simulink model "day3_TuNT54"  (R2017b)
settings: Solver=FixedStepAuto  StartTime=0.0  StopTime=1  FixedStep=0.002  RelTol=1e-3
libraries: simulink x5
settings Model: Creator=Admin  LastModifiedBy=Admin

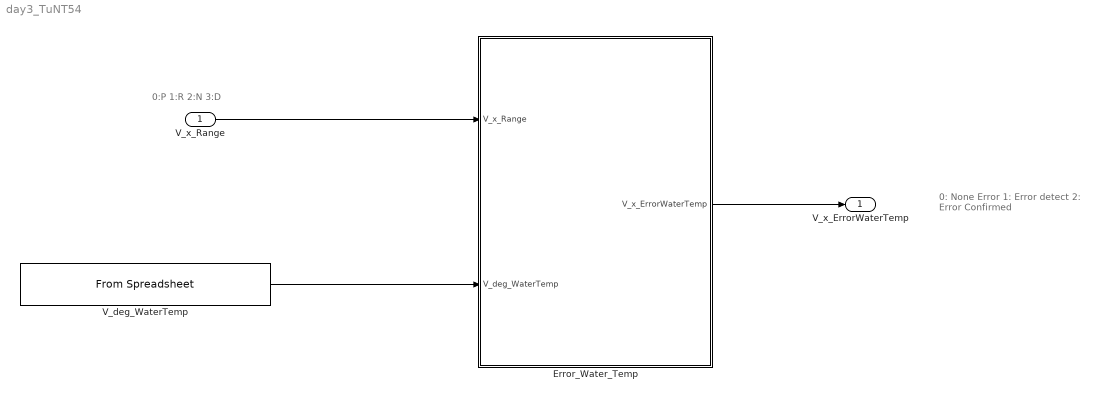
== system day3_TuNT54 ==
  note: 0: None Error
      | 1: Error detect
      | 2: Error Confirmed
  note: 0:P
      | 1:R
      | 2:N
      | 3:D
  V_x_Range : Inport
  Error_Water_Temp : Subsystem
  V_deg_WaterTemp : FromSpreadsheet  FileName=Data.xlsx
  V_x_ErrorWaterTemp : Outport
  wires:
  V_deg_WaterTemp/1 -> Error_Water_Temp/2(V_deg_WaterTemp)
  Error_Water_Temp/1(V_x_ErrorWaterTemp) -> V_x_ErrorWaterTemp/1
  V_x_Range/1 -> Error_Water_Temp/1(V_x_Range)

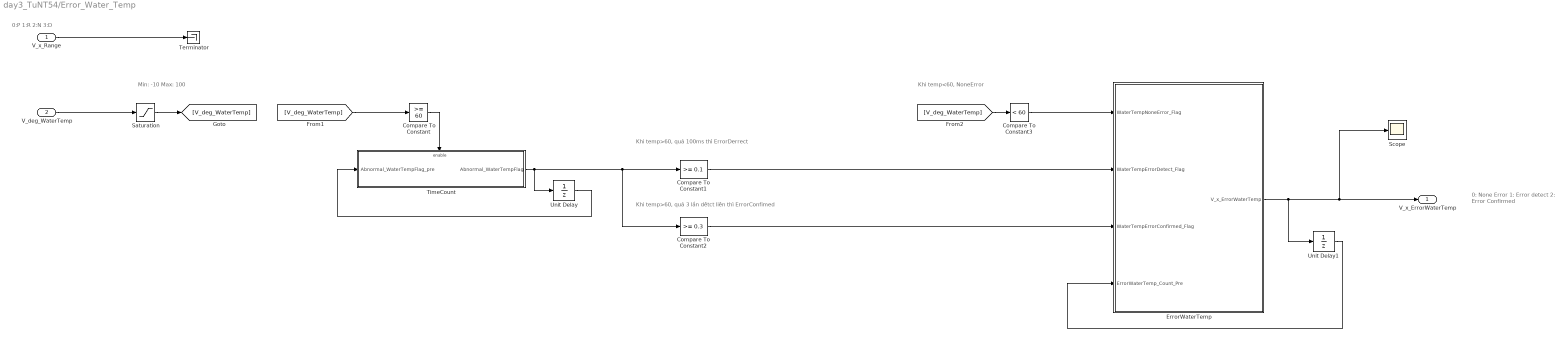
== system day3_TuNT54/Error_Water_Temp ==
  note: 0:P
      | 1:R
      | 2:N
      | 3:D
  note: 0: None Error
      | 1: Error detect
      | 2: Error Confirmed
  note: Min: -10
      | Max: 100
  note: Khi temp>60, quá 100ms thì ErrorDerrect
  note: Khi temp>60, quá 3 lần dêtct liên thì ErrorConfimed
  note: Khi temp<60, NoneError
  V_x_Range : Inport
  V_deg_WaterTemp : Inport  Port=2
  Compare To Constant : simulink/Logic and Bit Operations/Compare To Constant  relop=>=  const=60  OutDataTypeStr=boolean
  Compare To Constant1 : simulink/Logic and Bit Operations/Compare To Constant  relop=>=  const=0.1  OutDataTypeStr=boolean
  Compare To Constant2 : simulink/Logic and Bit Operations/Compare To Constant  relop=>=  const=0.3  OutDataTypeStr=boolean
  Compare To Constant3 : simulink/Logic and Bit Operations/Compare To Constant  relop=<  const=60  OutDataTypeStr=boolean
  ErrorWaterTemp : Subsystem
  Saturation : Saturate  UpperLimit=100  LowerLimit=-10
  Scope : Scope
  Terminator : Terminator
  TimeCount : Subsystem  TreatAsAtomicUnit=on
  Unit Delay : UnitDelay  SampleTime=-1
  Unit Delay1 : UnitDelay  SampleTime=-1
  V_x_ErrorWaterTemp : Outport
  wires:
  Unit Delay1/1 -> ErrorWaterTemp/4(ErrorWaterTemp_Count_Pre)
  TimeCount/1(Abnormal_WaterTempFlag) -> Compare To Constant2/1, Compare To Constant1/1, Unit Delay/1
  Compare To Constant3/1 -> ErrorWaterTemp/1(WaterTempNoneError_Flag)
  Compare To Constant/1 -> TimeCount/Enable
  Unit Delay/1 -> TimeCount/1(Abnormal_WaterTempFlag_pre)
  V_deg_WaterTemp/1 -> Saturation/1
  V_x_Range/1 -> Terminator/1
  ErrorWaterTemp/1(V_x_ErrorWaterTemp) -> Scope/1, V_x_ErrorWaterTemp/1, Unit Delay1/1
  Saturation/1 -> [V_deg_WaterTemp]
  [V_deg_WaterTemp] -> Compare To Constant/1
  [V_deg_WaterTemp] -> Compare To Constant3/1
  Compare To Constant1/1 -> ErrorWaterTemp/2(WaterTempErrorDetect_Flag)
  Compare To Constant2/1 -> ErrorWaterTemp/3(WaterTempErrorConfirmed_Flag)

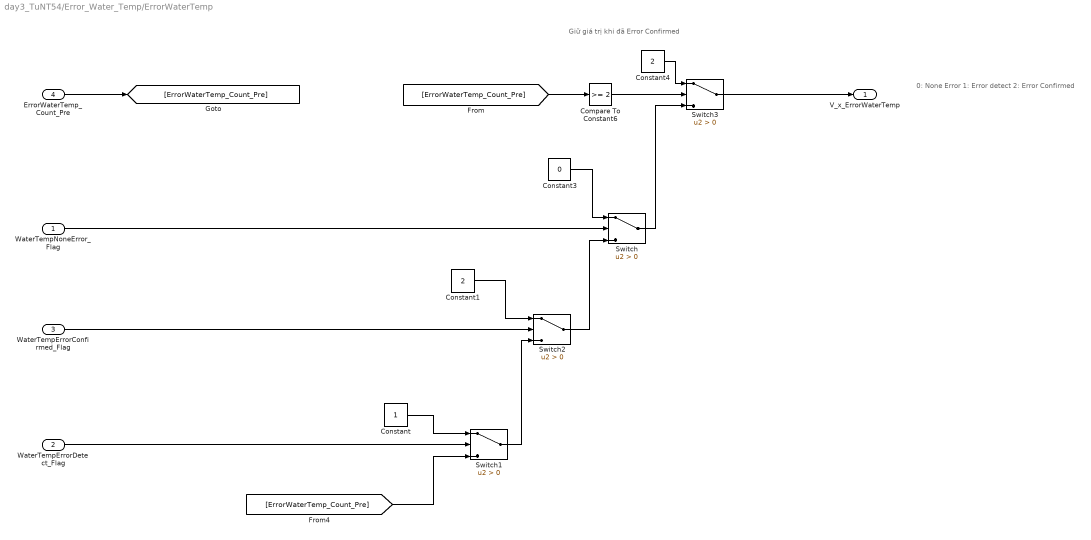
== system day3_TuNT54/Error_Water_Temp/ErrorWaterTemp ==
  note: 0: None Error
      | 1: Error detect
      | 2: Error Confirmed
  note: Giữ giá trị khi đã Error Confirmed
  WaterTempNoneError_Flag : Inport
  WaterTempErrorDetect_Flag : Inport  Port=2
  WaterTempErrorConfirmed_Flag : Inport  Port=3
  ErrorWaterTemp_Count_Pre : Inport  Port=4
  Compare To Constant6 : simulink/Logic and Bit Operations/Compare To Constant  relop=>=  const=2  OutDataTypeStr=boolean
  Constant : Constant
  Constant1 : Constant  Value=2
  Constant3 : Constant  Value=0
  Constant4 : Constant  Value=2
  Switch{,1..3} (4 alike) : Switch  Criteria=u2 > Threshold
  V_x_ErrorWaterTemp : Outport
  wires:
  Switch3/1 -> V_x_ErrorWaterTemp/1
  Constant4/1 -> Switch3/1
  WaterTempNoneError_Flag/1 -> Switch/2
  Constant3/1 -> Switch/1
  Switch/1 -> Switch3/3
  Compare To Constant6/1 -> Switch3/2
  WaterTempErrorDetect_Flag/1 -> Switch1/2
  ErrorWaterTemp_Count_Pre/1 -> [ErrorWaterTemp_Count_Pre]
  [ErrorWaterTemp_Count_Pre] -> Compare To Constant6/1
  [ErrorWaterTemp_Count_Pre] -> Switch1/3
  Constant/1 -> Switch1/1
  WaterTempErrorConfirmed_Flag/1 -> Switch2/2
  Switch1/1 -> Switch2/3
  Switch2/1 -> Switch/3
  Constant1/1 -> Switch2/1

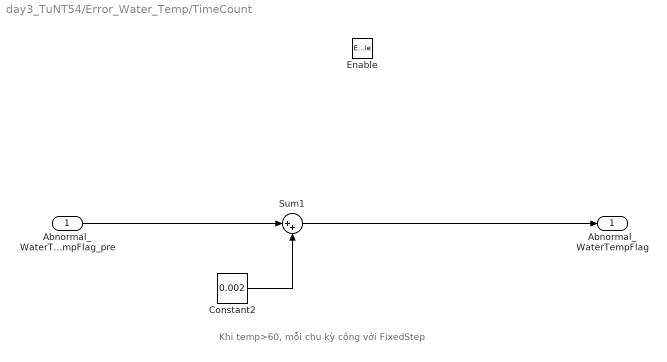
== system day3_TuNT54/Error_Water_Temp/TimeCount ==
  note: Khi temp>60, mỗi chu kỳ cộng với FixedStep
  Abnormal_WaterTempFlag_pre : Inport
  Enable : EnablePort  StatesWhenEnabling=reset
  Constant2 : Constant  Value=0.002
  Sum1 : Sum  Inputs=|++
  Abnormal_WaterTempFlag : Outport  OutputWhenDisabled=reset  InitialOutput=0
  wires:
  Sum1/1 -> Abnormal_WaterTempFlag/1
  Abnormal_WaterTempFlag_pre/1 -> Sum1/1
  Constant2/1 -> Sum1/2
